simulink model "model"  (R2021a)
settings: Solver=VariableStepAuto  StartTime=0.0  StopTime=10.0  RelTol=1e-3
settings Model: Creator=amejiyopakapak  LastModifiedBy=amejiyopakapak

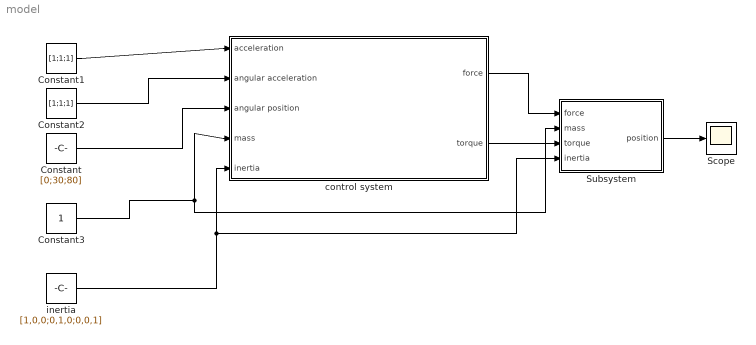
== system model ==
  Constant : Constant  Value=[0;30;80]  VectorParams1D=off
  Constant1 : Constant  Value=[1;1;1]  VectorParams1D=off
  Constant2 : Constant  Value=[1;1;1]  VectorParams1D=off
  Constant3 : Constant
  Scope : Scope
  Subsystem : Subsystem
  control system : Subsystem
  inertia : Constant  Value=[1,0,0;0,1,0;0,0,1]  VectorParams1D=off
  wires:
  Constant/1 -> control system/3(angular position)
  Constant1/1 -> control system/1(acceleration)
  Constant2/1 -> control system/2(angular acceleration)
  Constant3/1 -> control system/4(mass), Subsystem/2(mass)
  inertia/1 -> Subsystem/4(inertia), control system/5(inertia)
  control system/1(force) -> Subsystem/1(force)
  control system/2(torque) -> Subsystem/3(torque)
  Subsystem/1(position) -> Scope/1

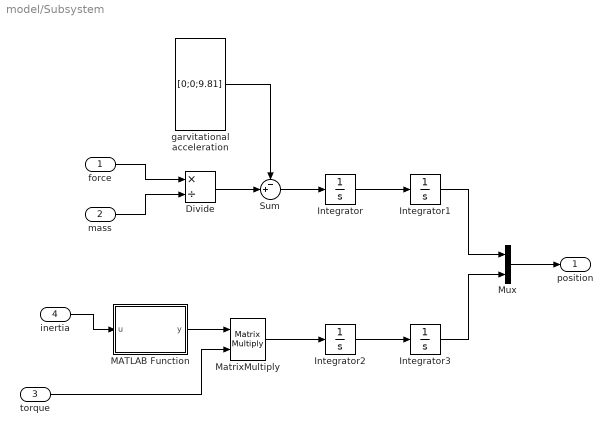
== system model/Subsystem ==
  force : Inport
  mass : Inport  Port=2
  torque : Inport  Port=3
  inertia : Inport  Port=4
  Divide : Product  Inputs=*/
  Integrator{,1..3} (4 alike) : Integrator
  MATLAB Function : MATLAB Function  TreatAsAtomicUnit=on
  MatrixMultiply : Product  Multiplication=Matrix(*)
  Mux : Mux  Inputs=2
  Sum : Sum  Inputs=-+|
  garvitational acceleration : Constant  Value=[0;0;9.81]  VectorParams1D=off
  position : Outport
  wires:
  Mux/1 -> position/1
  garvitational acceleration/1 -> Sum/1
  MatrixMultiply/1 -> Integrator2/1
  MATLAB Function/1(y) -> MatrixMultiply/1
  torque/1 -> MatrixMultiply/2
  Sum/1 -> Integrator/1
  Integrator1/1 -> Mux/1
  Divide/1 -> Sum/2
  Integrator2/1 -> Integrator3/1
  Integrator3/1 -> Mux/2
  force/1 -> Divide/1
  mass/1 -> Divide/2
  inertia/1 -> MATLAB Function/1(u)
  Integrator/1 -> Integrator1/1

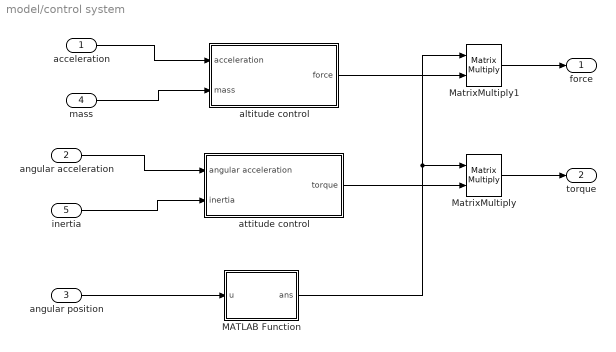
== system model/control system ==
  acceleration : Inport
  angular acceleration : Inport  Port=2
  angular position : Inport  Port=3
  mass : Inport  Port=4
  inertia : Inport  Port=5
  MATLAB Function : MATLAB Function  TreatAsAtomicUnit=on
  MatrixMultiply : Product  Multiplication=Matrix(*)
  MatrixMultiply1 : Product  Multiplication=Matrix(*)
  altitude control : Subsystem
  attitude control : Subsystem
  force : Outport
  torque : Outport  Port=2
  wires:
  acceleration/1 -> altitude control/1(acceleration)
  angular acceleration/1 -> attitude control/1(angular acceleration)
  angular position/1 -> MATLAB Function/1(u)
  MATLAB Function/1(ans) -> MatrixMultiply1/1, MatrixMultiply/1
  MatrixMultiply/1 -> torque/1
  attitude control/1(torque) -> MatrixMultiply/2
  MatrixMultiply1/1 -> force/1
  altitude control/1(force) -> MatrixMultiply1/2
  inertia/1 -> attitude control/2(inertia)
  mass/1 -> altitude control/2(mass)

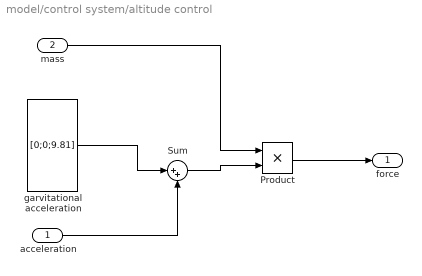
== system model/control system/altitude control ==
  acceleration : Inport
  mass : Inport  Port=2
  Product : Product
  Sum : Sum  Inputs=|++
  garvitational acceleration : Constant  Value=[0;0;9.81]  VectorParams1D=off
  force : Outport
  wires:
  Sum/1 -> Product/2
  garvitational acceleration/1 -> Sum/1
  Product/1 -> force/1
  acceleration/1 -> Sum/2
  mass/1 -> Product/1

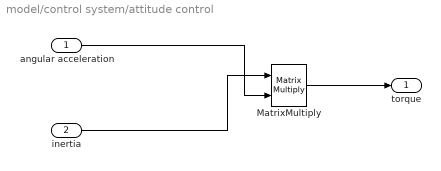
== system model/control system/attitude control ==
  angular acceleration : Inport
  inertia : Inport  Port=2
  MatrixMultiply : Product  Multiplication=Matrix(*)
  torque : Outport
  wires:
  MatrixMultiply/1 -> torque/1
  angular acceleration/1 -> MatrixMultiply/2
  inertia/1 -> MatrixMultiply/1

== matlab function model/control system/MATLAB Function ==
  data: u input; ans output
function ans = rotationMatrix(u)
    r = u(1);
    p = u(2);
    y = u(3);
    ans = [cos(y)*cos(r), (-sin(y)*cos(r)) + (cos(y)*sin(p)*sin(r)), sin(y)*sin(r) + cos(y)*sin(p)*cos(r);sin(y)*cos(p), cos(y)*cos(r)+sin(y)*sin(p)*sin(r), -cos(y)*sin(r) + sin(y)*sin(p)*cos(r);-sin(p),cos(p)*sin(r),cos(p)*cos(r)];
ans;

== matlab function model/Subsystem/MATLAB Function ==
  data: u input; y output
function y = inverseMatrix(u)

y = inv(u);
